simulink model "newQuatLib"  (R2015a)
settings: Solver=ode45  StartTime=0.0  StopTime=10.0  RelTol=1e-3
undefined symbols (not defined in the file): randquatiso
libraries: simulink x1
(part 1 of 2)
settings Model: Creator=lagadec  LastModifiedBy=lagadec
settings DebuggingCC: UnderspecifiedInitializationDetection=Classic  MergeDetectMultiDrivingBlocksExec=none  SolverPrmCheckMsg=warning

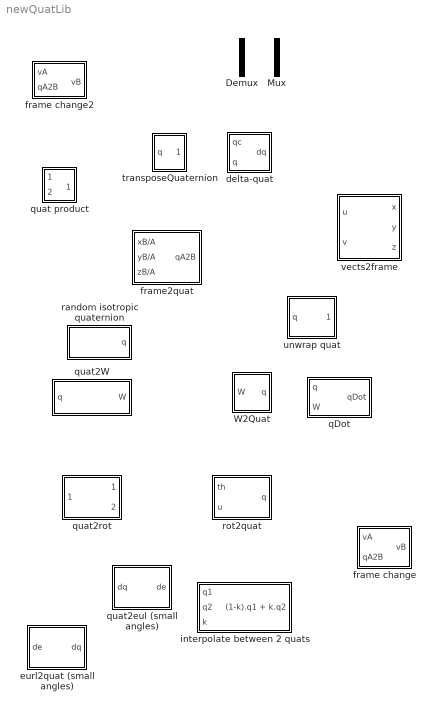
== system newQuatLib ==
  Demux : Demux  Outputs=[1 3]
  Mux : Mux  Inputs=2
  W2Quat : Subsystem  Tag=40  mask(W2Quat){q_init=randquatiso(1)}
      mask prompts: q_init "Initial quaternion"
      mask help:
      | Compute attitude quaternion from instantaneous angular velocity of the rigid body expressed in body frame :
      | w = [p q r]'
      |
      | K. Lagadec 1998
      mask Help: eval('AstrolibHelp');
      mask Display: disp('\Omega=\intq','texmode','on')
  delta-quat : Subsystem  mask(deltaQuaternion){}
      mask help:
      | Computes the 'difference' between 2 attitudes, i.e. the quaternion Dq such that:
      | dq = qc'*q
      | (analogous to dtheta = theta_c - theta for 1-d angles)
  eurl2quat (small angles) : Subsystem  mask(Small euler angles error to small quat){}
      mask help: dq = [1; e(1)/2 ; e(2)/2 ; e(3)/2]
  frame change : Subsystem  mask(Frame change){inLabel=I, outLabel=B}
      mask prompts: inLabel "Label for initial frame"; outLabel "Label for target frame"
      mask help: Express input vector in frame B, using the quaternion describing the rotation from frame A to frame B.
      mask Display:
      | port_label('input',1,['v',inLabel]);
      | port_label('output',1,['v',outLabel]);
      | port_label('input',2,['q',inLabel,'2',outLabel]);
  frame change2 : Subsystem  mask(Frame change){inLabel=I, outLabel=T, flipQuat=off}
      mask prompts: inLabel "Label for initial frame"; outLabel "Label for target frame"; flipQuat "Transpose input quaternion"
      mask help: Express input vector in target frame, using the quaternion describing the rotation from origin frame to target frame.
      mask init:
      | if flipQuat
      |     qLabel = ['q',outLabel,'2',inLabel];
      | else
      |     qLabel = ['q',inLabel,'2',outLabel];
      | end
      mask Display:
      | port_label('input',1,['v',inLabel]);
      | port_label('output',1,['v',outLabel]);
      | port_label('input',2,qLabel);
  frame2quat : Subsystem  mask(Compute quaternion from 3 orthogonal unit vectors){Alabel=I, Blabel=B}
      mask prompts: Alabel "Label for origin frame"; Blabel "Label for target frame"
      mask help: Determines the attitude quaternion representing the rotation which transforms the origin frame into the target frame, from the unit vectors of target frame expressed in origin frame.
      mask Display:
      | port_label('input',1,['x',Blabel,'/',Alabel]);
      | port_label('input',2,['y',Blabel,'/',Alabel]);
      | port_label('input',3,['z',Blabel,'/',Alabel]);
      | port_label('output',1,['q',Alabel,'2',Blabel]);
  interpolate between 2 quats : Subsystem
  qDot : Subsystem  Tag=40  mask(W2dqdt){}
      mask help:
      | Compute quaternion derivative from instantaneous angular velocity of the rigid body expressed in body frame :
      | dq/dt = 0.5*q*W
      | K. Lagadec 1998
  quat product : Subsystem
      mask Display:
      | plot(0.5+cos(linspace(0,2*pi,65))*0.25,0.5+sin(linspace(0,2*pi,65))*0.25);
      | plot([.32 .68],[.32 .68]);
      | plot([.68 .32],[.32 .68]);
  quat2W : Subsystem  mask(Quaternion differentiation){Ts=1}
      mask prompts: Ts "Sample time"
      mask help:
      | Compute angular velocity vector by differentiating the attitude quaternion :
      |
      | W = 2*q'*dq/dt
      mask Display: disp('\Omega~2q''(\deltaq/\deltat)','texmode','on')
  quat2eul (small angles) : Subsystem  mask(Small quat error to small angles error){}
      mask help:
      | [dphi,dtheta,dpsi] = u*dTheta
      | where
      | dq = [cos(dTheta/2); u*sin(dTheta/2)]
  quat2rot : Subsystem  mask(Find axis and angle from quaternion){Alabel=I, Blabel=B}
      mask prompts: Alabel "Label for origin frame"; Blabel "Label for target frame"
      mask help: Extracts the axis (unit vector) and angle (rad) of the rotation from origin frame to target frame, from the quaternion representing that rotation
      mask Display:
      | port_label('input',1,['q',Alabel,'2',Blabel]);
      | port_label('output',1,['th_',Alabel,'2',Blabel]);
      | port_label('output',2,['u_',Alabel]);
  random isotropic quaternion : Subsystem  mask(Random quaternion (isotropic)){Ts=1}
      mask prompts: Ts "Sample time"
      mask help:
      | Simple random isotropic quaternion, made by normalizing a 4-vector with gaussian random components.
      | (because quaternion space is equivalent to the 3-sphere (unit sphere in 4D)).
      |
      | K. Lagadec, 2016
      mask Display: disp('randquat')
  rot2quat : Subsystem  mask(Rotation to quaternion){Alabel=I, Blabel=B}
      mask prompts: Alabel "Label for origin frame"; Blabel "Label for target frame"
      mask help:
      | Computes quaternion from elementary components: rotation axis u and rotation angle theta
      | by convention, norm(u) = 1
      | q(1) = cos(theta/2)
      | q(2) = u(1)*sin(theta/2)
      | q(3) = u(2)*sin(theta/2)
      | q(4) = u(3)*sin(theta/2)
      |
      | K. Lagadec 2000
      mask Display:
      | port_label('output',1,['q',Alabel,'2',Blabel]);
      | port_label('input',1,['th_',Alabel,'2',Blabel]);
      | port_label('input',2,['u_',Alabel]);
  transposeQuaternion : Subsystem  mask(transposeQuaternion){}
      mask help:
      | Compute the transpose (inverse or conjugate) of the input quaternion
      |
      | Inputs:
      |   q     Quaternion
      |
      | Outputs:
      |   qt     Transpose of the input quaternion
      mask Help: eval('starDoc simulink/transposeQuaternion');
      mask Display: disp('q''');
  unwrap quat : Subsystem  mask(Unwrap quaternion){}
      mask help: Avoid sudden jumps q => -q when both quaternions are equivalent. Produces smooth quaternion output unless there are real discontinuities in attitude.
  vects2frame : Subsystem  mask(vects2frame){axisOrder=yx}
      mask prompts: axisOrder "Axes defined by u and v"
      mask help:
      | Construct a right-handed orthogonal frame from 2 directions
      | The first direction defines one of the target axes
      | The second direction defines another axis
      | If the two directions are not perpendicular, the first one has priority.
      | If the two directions are parallel, there will be a div by zero.
      |
      | Input vectors are normalized inside the mask
      mask init:
      | switch axisOrder
      |     case 'xy'
      |         order_i = [1 2 3];
      |         sign_i = [1 1 1];
      |     case 'xz'
      |         order_i = [1 3 2];
      |         sign_i = [1 -1 1];
      |     case 'yx'
      |         order_i = [2 1 3];
      |         sign_i = [1 1 -1];
      |     case 'yz'
      |         order_i = [3 1 2];
      |         sign_i = [1 1 1];
      |     case 'zx'
      |         order_i = [2 3 1];
      |         sign_i = [1 1 1];
      |     case 'zy'
      |         order_i = [3 2 1];
      |         sign_i = [-1 1 1];
      | end
      mask TypeOptions axisOrder: xy | xz | yx | yz | zx | zy
      mask Display:
      | port_label('input',1,axisOrder(1));
      | port_label('input',2,axisOrder(2));
      | 
      | port_label('output',1,'x');
      | port_label('output',2,'y');
      | port_label('output',3,'z');

== system newQuatLib/W2Quat ==
  note: q_dot = 1/2 q.W
  W : Inport  PortDimensions=3
  Constant : Constant  Value=0
  Gain : Gain  Gain=1/2  SaturateOnIntegerOverflow=on  OutDataTypeStr=Inherit: Same as input  ParamDataTypeStr=Inherit: Same as input
  Integrator : Integrator  InitialCondition=q_init
  Normalization : Subsystem  Tag=74
      mask help:
      | normalizes a vector, so that the output is a unit vector.
      | y = u/||u||
      mask Help: eval('AstrolibHelp');
      mask Display: disp('X/||X||');
  Transform into quaternion : Mux  Inputs=2
  quat product : Subsystem
      mask Display:
      | plot(0.5+cos(linspace(0,2*pi,65))*0.3,0.5+sin(linspace(0,2*pi,65))*0.3);
      | plot([.29 .71],[.29 .71]);
      | plot([.71 .29],[.29 .71]);
  q : Outport  PortDimensions=4  InitialOutput=0
  wires:
  quat product/1(q1*q2) -> Gain/1
  Gain/1 -> Integrator/1  "q_dot"
  Integrator/1 -> Normalization/1(X)
  Normalization/1(X/||X||) -> quat product/1(q1), q/1
  Transform into quaternion/1 -> quat product/2(q2)
  W/1 -> Transform into quaternion/2
  Constant/1 -> Transform into quaternion/1

== system newQuatLib/delta-quat ==
  qc : Inport  PortDimensions=4
  q : Inport  Port=2  PortDimensions=4
  quat product : Subsystem
      mask Display:
      | plot(0.5+cos(linspace(0,2*pi,65))*0.3,0.5+sin(linspace(0,2*pi,65))*0.3);
      | plot([.29 .71],[.29 .71]);
      | plot([.71 .29],[.29 .71]);
  transposeQuaternion : Subsystem  mask(transposeQuaternion){}
      mask help:
      | Compute the transpose (inverse or conjugate) of the input quaternion
      |
      | Inputs:
      |   q     Quaternion
      |
      | Outputs:
      |   qt     Transpose of the input quaternion
      mask Help: eval('starDoc simulink/transposeQuaternion');
      mask Display: disp('q''');
  dq : Outport  PortDimensions=4
  wires:
  q/1 -> quat product/2(q2)
  quat product/1(q1*q2) -> dq/1
  qc/1 -> transposeQuaternion/1(q)
  transposeQuaternion/1(q') -> quat product/1(q1)  "qA2B"

== system newQuatLib/eurl2quat (small angles) ==
  de : Inport  PortDimensions=3
  Mux : Mux  Inputs=2
  Normalization : Subsystem  Tag=74
      mask help:
      | normalizes a vector, so that the output is a unit vector.
      | y = u/||u||
      mask Help: eval('AstrolibHelp');
      mask Display: disp('X/||X||');
  half : Gain  Gain=0.5
  scalar : Constant
  dq : Outport  PortDimensions=4
  wires:
  de/1 -> half/1
  half/1 -> Mux/2
  scalar/1 -> Mux/1
  Mux/1 -> Normalization/1(X)
  Normalization/1(X/||X||) -> dq/1

== system newQuatLib/frame change ==
  vA : Inport
  qA2B : Inport  Port=2
  Constant : Constant
  Demux : Demux  Outputs=[1 3]
  Mux : Mux  Inputs=2
  Product : Product  Inputs=/*  SaturateOnIntegerOverflow=on  OutDataTypeStr=Inherit: Same as first input
  quat product : Subsystem
      mask Display:
      | plot(0.5+cos(linspace(0,2*pi,65))*0.3,0.5+sin(linspace(0,2*pi,65))*0.3);
      | plot([.29 .71],[.29 .71]);
      | plot([.71 .29],[.29 .71]);
  quat product1 : Subsystem
      mask Display:
      | plot(0.5+cos(linspace(0,2*pi,65))*0.3,0.5+sin(linspace(0,2*pi,65))*0.3);
      | plot([.29 .71],[.29 .71]);
      | plot([.71 .29],[.29 .71]);
  transposeQuaternion : Subsystem  mask(transposeQuaternion){}
      mask help:
      | Compute the transpose (inverse or conjugate) of the input quaternion
      |
      | Inputs:
      |   q     Quaternion
      |
      | Outputs:
      |   qt     Transpose of the input quaternion
      mask Help: eval('starDoc simulink/transposeQuaternion');
      mask Display: disp('q''');
  vB : Outport
  wires:
  Product/1 -> vB/1
  quat product1/1(q1*q2) -> Demux/1
  quat product/1(q1*q2) -> quat product1/1(q1)
  Mux/1 -> quat product/2(q2)
  transposeQuaternion/1(q') -> quat product/1(q1)
  qA2B/1 -> quat product1/2(q2), transposeQuaternion/1(q)
  vA/1 -> Mux/2
  Constant/1 -> Mux/1
  Demux/1 -> Product/1
  Demux/2 -> Product/2

== system newQuatLib/frame change2 ==
  vA : Inport  PortDimensions=3
  qA2B : Inport  Port=2  PortDimensions=4
  Constant : Constant
  Constant1 : Constant  Value=not(flipQuat)
  Constant2 : Constant  Value=flipQuat
  Demux : Demux  Outputs=[1 3]
  Mux : Mux  Inputs=2
  Product : Product  Inputs=/*  SaturateOnIntegerOverflow=on  OutDataTypeStr=Inherit: Same as first input
  Switch : Switch  Criteria=u2 ~= 0
  Switch1 : Switch  Criteria=u2 ~= 0
  quat product : Subsystem
      mask Display:
      | plot(0.5+cos(linspace(0,2*pi,65))*0.3,0.5+sin(linspace(0,2*pi,65))*0.3);
      | plot([.29 .71],[.29 .71]);
      | plot([.71 .29],[.29 .71]);
  quat product1 : Subsystem
      mask Display:
      | plot(0.5+cos(linspace(0,2*pi,65))*0.3,0.5+sin(linspace(0,2*pi,65))*0.3);
      | plot([.29 .71],[.29 .71]);
      | plot([.71 .29],[.29 .71]);
  transposeQuaternion : Subsystem  mask(transposeQuaternion){}
      mask help:
      | Compute the transpose (inverse or conjugate) of the input quaternion
      |
      | Inputs:
      |   q     Quaternion
      |
      | Outputs:
      |   qt     Transpose of the input quaternion
      mask Help: eval('starDoc simulink/transposeQuaternion');
      mask Display: disp('q''');
  vB : Outport  PortDimensions=3
  wires:
  Demux/2 -> Product/2
  Demux/1 -> Product/1
  Constant/1 -> Mux/1
  vA/1 -> Mux/2
  qA2B/1 -> transposeQuaternion/1(q), Switch/3, Switch1/3
  transposeQuaternion/1(q') -> Switch1/1, Switch/1
  Mux/1 -> quat product/2(q2)
  quat product/1(q1*q2) -> quat product1/1(q1)
  quat product1/1(q1*q2) -> Demux/1
  Product/1 -> vB/1
  Constant1/1 -> Switch/2
  Switch/1 -> quat product/1(q1)
  Constant2/1 -> Switch1/2
  Switch1/1 -> quat product1/2(q2)

== system newQuatLib/frame2quat ==
  xB/A : Inport  PortDimensions=3
  yB/A : Inport  Port=2  PortDimensions=3
  zB/A : Inport  Port=3  PortDimensions=3
  MATLAB Function : MATLAB Function  TreatAsAtomicUnit=on
  qA2B : Outport  PortDimensions=4
  wires:
  xB/A/1 -> MATLAB Function/1(xB)
  yB/A/1 -> MATLAB Function/2(yB)
  zB/A/1 -> MATLAB Function/3(zB)
  MATLAB Function/1(qA2B) -> qA2B/1

== system newQuatLib/interpolate between 2 quats ==
  q1 : Inport
  q2 : Inport  Port=2
  k : Inport  Port=3
  MATLAB Function : MATLAB Function  TreatAsAtomicUnit=on
  (1-k).q1 + k.q2 : Outport
  wires:
  MATLAB Function/1(qi) -> (1-k).q1 + k.q2/1
  q2/1 -> MATLAB Function/2(q2)
  q1/1 -> MATLAB Function/1(q1)
  k/1 -> MATLAB Function/3(k)

== system newQuatLib/qDot ==
  note: q_dot = 1/2 q.W
  q : Inport  PortDimensions=4
  W : Inport  Port=2  PortDimensions=3
  Constant : Constant  Value=0
  Gain : Gain  Gain=1/2  SaturateOnIntegerOverflow=on  OutDataTypeStr=Inherit: Same as input  ParamDataTypeStr=Inherit: Same as input
  Transform into quaternion : Mux  Inputs=2
  quat product : Subsystem
      mask Display:
      | plot(0.5+cos(linspace(0,2*pi,65))*0.3,0.5+sin(linspace(0,2*pi,65))*0.3);
      | plot([.29 .71],[.29 .71]);
      | plot([.71 .29],[.29 .71]);
  qDot : Outport  PortDimensions=4  InitialOutput=0
  wires:
  Constant/1 -> Transform into quaternion/1
  W/1 -> Transform into quaternion/2
  Transform into quaternion/1 -> quat product/2(q2)
  quat product/1(q1*q2) -> Gain/1
  Gain/1 -> qDot/1  "q_dot"
  q/1 -> quat product/1(q1)

== system newQuatLib/quat product ==
  q1 : Inport  PortDimensions=4
  q2 : Inport  Port=2  PortDimensions=4
  Cross Product : Subsystem  Tag=68  mask(CrossProduct){}
      mask help: Compute the cross product of two 3-vectors : y = u1 x u2
      mask Display:
      | plot([.4 .6],[.4 .6]);
      | plot([.6 .4],[.4 .6]);
  Demux : Demux  Outputs=[1 3]
  Demux1 : Demux  Outputs=[1 3]
  Dot Product : DotProduct  InputSameDT=on  OutDataTypeStr=Inherit: Inherit via internal rule
  Mux : Mux  Inputs=2
  Product : Product  SaturateOnIntegerOverflow=on  OutDataTypeStr=Inherit: Same as first input
  Product1 : Product  SaturateOnIntegerOverflow=on  OutDataTypeStr=Inherit: Same as first input
  Product2 : Product  SaturateOnIntegerOverflow=on  OutDataTypeStr=Inherit: Same as first input
  Sum : Sum  Inputs=+++  SaturateOnIntegerOverflow=on
  Sum1 : Sum  Inputs=|+-  SaturateOnIntegerOverflow=on
  q1*q2 : Outport  PortDimensions=4
  wires:
  Demux/2 -> Product1/2, Cross Product/1(u1), Dot Product/2
  Demux/1 -> Product/1, Product2/1
  Demux1/1 -> Product1/1, Product2/2
  Demux1/2 -> Cross Product/2(u2), Product/2, Dot Product/1
  Cross Product/1(u1xu2) -> Sum/2
  Product/1 -> Sum/1
  Product1/1 -> Sum/3
  Sum/1 -> Mux/2  "vector"
  Product2/1 -> Sum1/1
  Dot Product/1 -> Sum1/2
  Sum1/1 -> Mux/1  "scalar"
  q1/1 -> Demux/1
  Mux/1 -> q1*q2/1
  q2/1 -> Demux1/1

== system newQuatLib/quat2W ==
  note: W = 2*q'*dq/dt
  q : Inport  PortDimensions=4  SampleTime=Ts
  Discrete Derivative : simulink/Discrete/Discrete Derivative  gainval=1.0  ICPrevScaledInput=0.0  InputProcessing=Inherited  OutMin=[]  OutMax=[]  OutDataType=fixdt(1, 16)  OutScaling=2^-10  DoSatur=off
  Selector : Selector  InputPortWidth=4  Indices=[2:4]
  quat product : Subsystem
      mask Display:
      | plot(0.5+cos(linspace(0,2*pi,65))*0.25,0.5+sin(linspace(0,2*pi,65))*0.25);
      | plot([.32 .68],[.32 .68]);
      | plot([.68 .32],[.32 .68]);
  times two : Gain  Gain=2
  transposeQuaternion : Subsystem  mask(transposeQuaternion){}
      mask help:
      | Compute the transpose (inverse or conjugate) of the input quaternion
      |
      | Inputs:
      |   q     Quaternion
      |
      | Outputs:
      |   qt     Transpose of the input quaternion
      mask Help: eval('starDoc simulink/transposeQuaternion');
      mask Display: disp('q''');
  unwrap quat : Subsystem  mask(Unwrap quaternion){}
      mask help: Avoid sudden jumps q => -q when both quaternions are equivalent. Produces smooth quaternion output unless there are real discontinuities in attitude.
  W : Outport  PortDimensions=3
  wires:
  q/1 -> unwrap quat/1(q)
  times two/1 -> W/1
  Selector/1 -> times two/1
  quat product/1(q1*q2) -> Selector/1
  Discrete Derivative/1 -> quat product/2(q2)  "scalar"
  unwrap quat/1(q_unw) -> Discrete Derivative/1, transposeQuaternion/1(q)
  transposeQuaternion/1(q') -> quat product/1(q1)

== system newQuatLib/quat2eul (small angles) ==
  dq : Inport  PortDimensions=4
  Demux : Demux  Outputs=[1 3]
  Gain : Gain  Gain=2
  manage quat sign : Switch  Criteria=u2 > Threshold
  take opposite : Gain  Gain=-1
  de : Outport  PortDimensions=3
  wires:
  Gain/1 -> de/1
  dq/1 -> Demux/1
  Demux/1 -> manage quat sign/2  "scalar"
  Demux/2 -> manage quat sign/1, take opposite/1
  take opposite/1 -> manage quat sign/3
  manage quat sign/1 -> Gain/1

== system newQuatLib/quat2rot ==
  q_AB : Inport  PortDimensions=4
  Constant : Constant
  Demux : Demux  Outputs=[1 3]
  Divide : Product  Inputs=***
  Divide1 : Product  Inputs=/
  Divide2 : Product  Inputs=**
  Gain : Gain  Gain=2
  Norm : Subsystem  mask(Norm){}
      mask help: Computes the norm of a vector : y = ||u||.
      mask Help: eval('AstrolibHelp');
      mask Display: disp('||X||');
  Sign : Signum  ZeroCross=off
  Switch : Switch  Criteria=u2 ~= 0  ZeroCross=off
  Trigonometric Function : Trigonometry  Operator=atan2
  angleB2A : Outport  PortDimensions=1
  vector_A : Outport  Port=2  PortDimensions=3
  wires:
  Sign/1 -> Divide2/2, Divide/1
  Divide2/1 -> Trigonometric Function/2
  Divide1/1 -> Divide/3
  q_AB/1 -> Demux/1
  Demux/1 -> Divide2/1, Sign/1
  Demux/2 -> Norm/1(X), Divide/2
  Trigonometric Function/1 -> Gain/1
  Gain/1 -> angleB2A/1
  Divide/1 -> vector_A/1
  Norm/1(||X||) -> Trigonometric Function/1, Switch/1, Switch/2
  Switch/1 -> Divide1/1
  Constant/1 -> Switch/3

== system newQuatLib/random isotropic quaternion ==
  Normalization : Subsystem  Tag=74
      mask help:
      | normalizes a vector, so that the output is a unit vector.
      | y = u/||u||
      mask Help: eval('AstrolibHelp');
      mask Display: disp('X/||X||');
  Random Number : RandomNumber  Seed=ceil(rand(4,1)*10000)  SampleTime=Ts
  q : Outport
  wires:
  Normalization/1(X/||X||) -> q/1  "q"
  Random Number/1 -> Normalization/1(X)

== system newQuatLib/rot2quat ==
  note: q(1) = cos(theta/2)
      | q(2) = u(1)*sin(theta/2)
      | q(3) = u(2)*sin(theta/2)
      | q(4) = u(3)*sin(theta/2)
  th : Inport  PortDimensions=1
  u : Inport  Port=2  PortDimensions=3
  Gain1 : Gain  Gain=1/2  SaturateOnIntegerOverflow=on  OutDataTypeStr=Inherit: Same as input  ParamDataTypeStr=Inherit: Same as input
  Mux : Mux  Inputs=2
  Product : Product  SaturateOnIntegerOverflow=on  RndMeth=Zero  InputSameDT=on  OutDataTypeStr=Inherit: Same as first input
  Trigonometric Function1 : Trigonometry
  Trigonometric Function2 : Trigonometry  Operator=cos
  q : Outport  PortDimensions=4
  wires:
  u/1 -> Product/2
  Trigonometric Function1/1 -> Product/1
  Mux/1 -> q/1
  Gain1/1 -> Trigonometric Function2/1, Trigonometric Function1/1
  th/1 -> Gain1/1
  Product/1 -> Mux/2
  Trigonometric Function2/1 -> Mux/1

== system newQuatLib/transposeQuaternion ==
  q : Inport  PortDimensions=4
  Gain1 : Gain  Gain=[1 -1 -1 -1]  SaturateOnIntegerOverflow=on  OutDataTypeStr=Inherit: Same as input  ParamDataTypeStr=Inherit: Same as input
  q' : Outport  PortDimensions=4
  wires:
  q/1 -> Gain1/1
  Gain1/1 -> q'/1

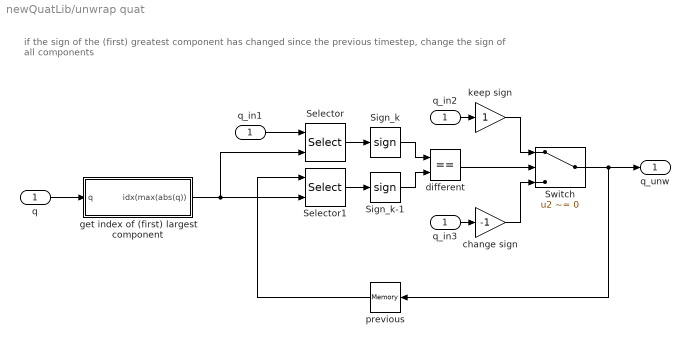
== system newQuatLib/unwrap quat ==
  note: if the sign of the (first) greatest component has changed since the previous timestep, change the sign of all components
  q : Inport
  Selector : Selector  InputPortWidth=4  IndexOptions=Index vector (port)  Indices=[1 3]
  Selector1 : Selector  InputPortWidth=4  IndexOptions=Index vector (port)  Indices=[1 3]
  Sign_k : Signum
  Sign_k-1 : Signum
  Switch : Switch  Criteria=u2 ~= 0
  change sign : Gain  Gain=-1
  different : RelationalOperator  Operator===  OutDataTypeStr=boolean
  get index of (first) largest component : Subsystem
  keep sign : Gain
  previous : Memory  X0=[1 1 1 1]  InheritSampleTime=on
  q_in1 : InportShadow
  q_in2 : InportShadow
  q_in3 : InportShadow
  q_unw : Outport
  wires:
  q_in3/1 -> change sign/1
  change sign/1 -> Switch/3
  keep sign/1 -> Switch/1
  q_in2/1 -> keep sign/1
  different/1 -> Switch/2
  Sign_k/1 -> different/1
  Sign_k-1/1 -> different/2
  Selector/1 -> Sign_k/1
  q_in1/1 -> Selector/1
  Switch/1 -> q_unw/1, previous/1
  previous/1 -> Selector1/1
  Selector1/1 -> Sign_k-1/1
  get index of (first) largest component/1(idx(max(abs(q))) -> Selector/2, Selector1/2
  q/1 -> get index of (first) largest component/1(q)

== system newQuatLib/vects2frame ==
  u : Inport  PortDimensions=3
  v : Inport  Port=2  PortDimensions=3
  Normalization : Subsystem  Tag=74
      mask help:
      | normalizes a vector, so that the output is a unit vector.
      | y = u/||u||
      mask Help: eval('AstrolibHelp');
      mask Display: disp('X/||X||');
  Normalization1 : Subsystem  Tag=74
      mask help:
      | normalizes a vector, so that the output is a unit vector.
      | y = u/||u||
      mask Help: eval('AstrolibHelp');
      mask Display: disp('X/||X||');
  cross product : Subsystem  Tag=68  mask(CrossProduct){}
      mask help: Compute the cross product of two 3-vectors : y = u1 x u2
      mask Display:
      | plot([.4 .6],[.4 .6]);
      | plot([.6 .4],[.4 .6]);
  cross product1 : Subsystem  Tag=68  mask(CrossProduct){}
      mask help: Compute the cross product of two 3-vectors : y = u1 x u2
      mask Display:
      | plot([.4 .6],[.4 .6]);
      | plot([.6 .4],[.4 .6]);
  reorder : Subsystem
  x : Outport
  y : Outport  Port=2
  z : Outport  Port=3
  wires:
  reorder/3(z) -> z/1
  reorder/2(y) -> y/1
  reorder/1(x) -> x/1
  cross product1/1(u1xu2) -> reorder/2((uxv)xu)
  Normalization1/1(X/||X||) -> cross product1/1(u1), reorder/3(uxv)
  cross product/1(u1xu2) -> Normalization1/1(X)
  v/1 -> cross product/2(u2)
  Normalization/1(X/||X||) -> cross product1/2(u2), reorder/1(u)
  u/1 -> Normalization/1(X), cross product/1(u1)

== system newQuatLib/W2Quat/Normalization ==
  X : Inport
      settings: AttributesFormatString=(#%<Tag>)
      mask Help: eval('AstrolibHelp');
  Constant : Constant
  Norm : Subsystem  mask(Norm){}
      mask help: Computes the norm of a vector : y = ||u||.
      settings: AttributesFormatString=(#%<Tag>)
      mask Help: eval('AstrolibHelp');
      mask Display: disp('||X||');
  Product : Product  Inputs=*/  RndMeth=Zero
  avoid div by zero : Switch  Criteria=u2 ~= 0
  x(1) = 1 : Assignment  DiagnosticForDimensions=Warning
  X/||X|| : Outport  InitialOutput=0
      settings: AttributesFormatString=(#%<Tag>)
      mask Help: eval('AstrolibHelp');
  wires:
  Norm/1(||X||) -> Product/2, avoid div by zero/2
  X/1 -> Product/1, x(1) = 1/1, Norm/1(X)
  Product/1 -> avoid div by zero/1
  avoid div by zero/1 -> X/||X||/1
  x(1) = 1/1 -> avoid div by zero/3
  Constant/1 -> x(1) = 1/2

== system newQuatLib/W2Quat/quat product ==
  q1 : Inport
  q2 : Inport  Port=2
  Cross Product : Subsystem  Tag=68  mask(CrossProduct){}
      mask help: Compute the cross product of two 3-vectors : y = u1 x u2
      mask Display:
      | plot([.4 .6],[.4 .6]);
      | plot([.6 .4],[.4 .6]);
  Demux : Demux  Outputs=[1 3]
  Demux1 : Demux  Outputs=[1 3]
  Dot Product : DotProduct  InputSameDT=on  OutDataTypeStr=Inherit: Inherit via internal rule
  Mux : Mux  Inputs=2
  Product : Product  SaturateOnIntegerOverflow=on  OutDataTypeStr=Inherit: Same as first input
  Product1 : Product  SaturateOnIntegerOverflow=on  OutDataTypeStr=Inherit: Same as first input
  Product2 : Product  SaturateOnIntegerOverflow=on  OutDataTypeStr=Inherit: Same as first input
  Sum : Sum  Inputs=+++  SaturateOnIntegerOverflow=on
  Sum1 : Sum  Inputs=|+-  SaturateOnIntegerOverflow=on
  q1*q2 : Outport
  wires:
  Demux/2 -> Product1/2, Cross Product/1(u1), Dot Product/2
  Demux/1 -> Product/1, Product2/1
  Demux1/1 -> Product1/1, Product2/2
  Demux1/2 -> Cross Product/2(u2), Product/2, Dot Product/1
  Cross Product/1(u1xu2) -> Sum/2
  Product/1 -> Sum/1
  Product1/1 -> Sum/3
  Sum/1 -> Mux/2  "vector"
  Product2/1 -> Sum1/1
  Dot Product/1 -> Sum1/2
  Sum1/1 -> Mux/1  "scalar"
  q1/1 -> Demux/1
  Mux/1 -> q1*q2/1
  q2/1 -> Demux1/1

== system newQuatLib/delta-quat/quat product ==
  q1 : Inport
  q2 : Inport  Port=2
  Cross Product : Subsystem  Tag=68  mask(CrossProduct){}
      mask help: Compute the cross product of two 3-vectors : y = u1 x u2
      mask Display:
      | plot([.4 .6],[.4 .6]);
      | plot([.6 .4],[.4 .6]);
  Demux : Demux  Outputs=[1 3]
  Demux1 : Demux  Outputs=[1 3]
  Dot Product : DotProduct  InputSameDT=on  OutDataTypeStr=Inherit: Inherit via internal rule
  Mux : Mux  Inputs=2
  Product : Product  SaturateOnIntegerOverflow=on  OutDataTypeStr=Inherit: Same as first input
  Product1 : Product  SaturateOnIntegerOverflow=on  OutDataTypeStr=Inherit: Same as first input
  Product2 : Product  SaturateOnIntegerOverflow=on  OutDataTypeStr=Inherit: Same as first input
  Sum : Sum  Inputs=+++  SaturateOnIntegerOverflow=on
  Sum1 : Sum  Inputs=|+-  SaturateOnIntegerOverflow=on
  q1*q2 : Outport
  wires:
  Demux/2 -> Product1/2, Cross Product/1(u1), Dot Product/2
  Demux/1 -> Product/1, Product2/1
  Demux1/1 -> Product1/1, Product2/2
  Demux1/2 -> Cross Product/2(u2), Product/2, Dot Product/1
  Cross Product/1(u1xu2) -> Sum/2
  Product/1 -> Sum/1
  Product1/1 -> Sum/3
  Sum/1 -> Mux/2  "vector"
  Product2/1 -> Sum1/1
  Dot Product/1 -> Sum1/2
  Sum1/1 -> Mux/1  "scalar"
  q1/1 -> Demux/1
  Mux/1 -> q1*q2/1
  q2/1 -> Demux1/1

== system newQuatLib/delta-quat/transposeQuaternion ==
  q : Inport
  Gain1 : Gain  Gain=[1 -1 -1 -1]  SaturateOnIntegerOverflow=on  OutDataTypeStr=Inherit: Same as input  ParamDataTypeStr=Inherit: Same as input
  q' : Outport
  wires:
  q/1 -> Gain1/1
  Gain1/1 -> q'/1

== system newQuatLib/eurl2quat (small angles)/Normalization ==
  X : Inport
      settings: AttributesFormatString=(#%<Tag>)
      mask Help: eval('AstrolibHelp');
  Constant : Constant
  Norm : Subsystem  mask(Norm){}
      mask help: Computes the norm of a vector : y = ||u||.
      settings: AttributesFormatString=(#%<Tag>)
      mask Help: eval('AstrolibHelp');
      mask Display: disp('||X||');
  Product : Product  Inputs=*/  RndMeth=Zero
  avoid div by zero : Switch  Criteria=u2 ~= 0
  x(1) = 1 : Assignment  DiagnosticForDimensions=Warning
  X/||X|| : Outport  InitialOutput=0
      settings: AttributesFormatString=(#%<Tag>)
      mask Help: eval('AstrolibHelp');
  wires:
  Norm/1(||X||) -> Product/2, avoid div by zero/2
  X/1 -> Product/1, x(1) = 1/1, Norm/1(X)
  Product/1 -> avoid div by zero/1
  avoid div by zero/1 -> X/||X||/1
  x(1) = 1/1 -> avoid div by zero/3
  Constant/1 -> x(1) = 1/2

== system newQuatLib/frame change/quat product ==
  q1 : Inport
  q2 : Inport  Port=2
  Cross Product : Subsystem  Tag=68  mask(CrossProduct){}
      mask help: Compute the cross product of two 3-vectors : y = u1 x u2
      mask Display:
      | plot([.4 .6],[.4 .6]);
      | plot([.6 .4],[.4 .6]);
  Demux : Demux  Outputs=[1 3]
  Demux1 : Demux  Outputs=[1 3]
  Dot Product : DotProduct  InputSameDT=on  OutDataTypeStr=Inherit: Inherit via internal rule
  Mux : Mux  Inputs=2
  Product : Product  SaturateOnIntegerOverflow=on  OutDataTypeStr=Inherit: Same as first input
  Product1 : Product  SaturateOnIntegerOverflow=on  OutDataTypeStr=Inherit: Same as first input
  Product2 : Product  SaturateOnIntegerOverflow=on  OutDataTypeStr=Inherit: Same as first input
  Sum : Sum  Inputs=+++  SaturateOnIntegerOverflow=on
  Sum1 : Sum  Inputs=|+-  SaturateOnIntegerOverflow=on
  q1*q2 : Outport
  wires:
  Demux/2 -> Product1/2, Cross Product/1(u1), Dot Product/2
  Demux/1 -> Product/1, Product2/1
  Demux1/1 -> Product1/1, Product2/2
  Demux1/2 -> Cross Product/2(u2), Product/2, Dot Product/1
  Cross Product/1(u1xu2) -> Sum/2
  Product/1 -> Sum/1
  Product1/1 -> Sum/3
  Sum/1 -> Mux/2  "vector"
  Product2/1 -> Sum1/1
  Dot Product/1 -> Sum1/2
  Sum1/1 -> Mux/1  "scalar"
  q1/1 -> Demux/1
  Mux/1 -> q1*q2/1
  q2/1 -> Demux1/1

== system newQuatLib/frame change/quat product1 ==
  q1 : Inport
  q2 : Inport  Port=2
  Cross Product : Subsystem  Tag=68  mask(CrossProduct){}
      mask help: Compute the cross product of two 3-vectors : y = u1 x u2
      mask Display:
      | plot([.4 .6],[.4 .6]);
      | plot([.6 .4],[.4 .6]);
  Demux : Demux  Outputs=[1 3]
  Demux1 : Demux  Outputs=[1 3]
  Dot Product : DotProduct  InputSameDT=on  OutDataTypeStr=Inherit: Inherit via internal rule
  Mux : Mux  Inputs=2
  Product : Product  SaturateOnIntegerOverflow=on  OutDataTypeStr=Inherit: Same as first input
  Product1 : Product  SaturateOnIntegerOverflow=on  OutDataTypeStr=Inherit: Same as first input
  Product2 : Product  SaturateOnIntegerOverflow=on  OutDataTypeStr=Inherit: Same as first input
  Sum : Sum  Inputs=+++  SaturateOnIntegerOverflow=on
  Sum1 : Sum  Inputs=|+-  SaturateOnIntegerOverflow=on
  q1*q2 : Outport
  wires:
  q2/1 -> Demux1/1
  Mux/1 -> q1*q2/1
  q1/1 -> Demux/1
  Sum1/1 -> Mux/1  "scalar"
  Dot Product/1 -> Sum1/2
  Product2/1 -> Sum1/1
  Sum/1 -> Mux/2  "vector"
  Product1/1 -> Sum/3
  Product/1 -> Sum/1
  Cross Product/1(u1xu2) -> Sum/2
  Demux1/2 -> Dot Product/1, Product/2, Cross Product/2(u2)
  Demux1/1 -> Product2/2, Product1/1
  Demux/1 -> Product2/1, Product/1
  Demux/2 -> Dot Product/2, Cross Product/1(u1), Product1/2

== system newQuatLib/frame change/transposeQuaternion ==
  q : Inport
  Gain1 : Gain  Gain=[1 -1 -1 -1]  SaturateOnIntegerOverflow=on  OutDataTypeStr=Inherit: Same as input  ParamDataTypeStr=Inherit: Same as input
  q' : Outport
  wires:
  q/1 -> Gain1/1
  Gain1/1 -> q'/1

== system newQuatLib/frame change2/quat product ==
  q1 : Inport
  q2 : Inport  Port=2
  Cross Product : Subsystem  Tag=68  mask(CrossProduct){}
      mask help: Compute the cross product of two 3-vectors : y = u1 x u2
      mask Display:
      | plot([.4 .6],[.4 .6]);
      | plot([.6 .4],[.4 .6]);
  Demux : Demux  Outputs=[1 3]
  Demux1 : Demux  Outputs=[1 3]
  Dot Product : DotProduct  InputSameDT=on  OutDataTypeStr=Inherit: Inherit via internal rule
  Mux : Mux  Inputs=2
  Product : Product  SaturateOnIntegerOverflow=on  OutDataTypeStr=Inherit: Same as first input
  Product1 : Product  SaturateOnIntegerOverflow=on  OutDataTypeStr=Inherit: Same as first input
  Product2 : Product  SaturateOnIntegerOverflow=on  OutDataTypeStr=Inherit: Same as first input
  Sum : Sum  Inputs=+++  SaturateOnIntegerOverflow=on
  Sum1 : Sum  Inputs=|+-  SaturateOnIntegerOverflow=on
  q1*q2 : Outport
  wires:
  q2/1 -> Demux1/1
  Mux/1 -> q1*q2/1
  q1/1 -> Demux/1
  Sum1/1 -> Mux/1  "scalar"
  Dot Product/1 -> Sum1/2
  Product2/1 -> Sum1/1
  Sum/1 -> Mux/2  "vector"
  Product1/1 -> Sum/3
  Product/1 -> Sum/1
  Cross Product/1(u1xu2) -> Sum/2
  Demux1/2 -> Dot Product/1, Product/2, Cross Product/2(u2)
  Demux1/1 -> Product2/2, Product1/1
  Demux/1 -> Product2/1, Product/1
  Demux/2 -> Dot Product/2, Cross Product/1(u1), Product1/2

== system newQuatLib/frame change2/quat product1 ==
  q1 : Inport
  q2 : Inport  Port=2
  Cross Product : Subsystem  Tag=68  mask(CrossProduct){}
      mask help: Compute the cross product of two 3-vectors : y = u1 x u2
      mask Display:
      | plot([.4 .6],[.4 .6]);
      | plot([.6 .4],[.4 .6]);
  Demux : Demux  Outputs=[1 3]
  Demux1 : Demux  Outputs=[1 3]
  Dot Product : DotProduct  InputSameDT=on  OutDataTypeStr=Inherit: Inherit via internal rule
  Mux : Mux  Inputs=2
  Product : Product  SaturateOnIntegerOverflow=on  OutDataTypeStr=Inherit: Same as first input
  Product1 : Product  SaturateOnIntegerOverflow=on  OutDataTypeStr=Inherit: Same as first input
  Product2 : Product  SaturateOnIntegerOverflow=on  OutDataTypeStr=Inherit: Same as first input
  Sum : Sum  Inputs=+++  SaturateOnIntegerOverflow=on
  Sum1 : Sum  Inputs=|+-  SaturateOnIntegerOverflow=on
  q1*q2 : Outport
  wires:
  Demux/2 -> Product1/2, Cross Product/1(u1), Dot Product/2
  Demux/1 -> Product/1, Product2/1
  Demux1/1 -> Product1/1, Product2/2
  Demux1/2 -> Cross Product/2(u2), Product/2, Dot Product/1
  Cross Product/1(u1xu2) -> Sum/2
  Product/1 -> Sum/1
  Product1/1 -> Sum/3
  Sum/1 -> Mux/2  "vector"
  Product2/1 -> Sum1/1
  Dot Product/1 -> Sum1/2
  Sum1/1 -> Mux/1  "scalar"
  q1/1 -> Demux/1
  Mux/1 -> q1*q2/1
  q2/1 -> Demux1/1

== system newQuatLib/frame change2/transposeQuaternion ==
  q : Inport
  Gain1 : Gain  Gain=[1 -1 -1 -1]  SaturateOnIntegerOverflow=on  OutDataTypeStr=Inherit: Same as input  ParamDataTypeStr=Inherit: Same as input
  q' : Outport
  wires:
  Gain1/1 -> q'/1
  q/1 -> Gain1/1

== system newQuatLib/qDot/quat product ==
  q1 : Inport
  q2 : Inport  Port=2
  Cross Product : Subsystem  Tag=68  mask(CrossProduct){}
      mask help: Compute the cross product of two 3-vectors : y = u1 x u2
      mask Display:
      | plot([.4 .6],[.4 .6]);
      | plot([.6 .4],[.4 .6]);
  Demux : Demux  Outputs=[1 3]
  Demux1 : Demux  Outputs=[1 3]
  Dot Product : DotProduct  InputSameDT=on  OutDataTypeStr=Inherit: Inherit via internal rule
  Mux : Mux  Inputs=2
  Product : Product  SaturateOnIntegerOverflow=on  OutDataTypeStr=Inherit: Same as first input
  Product1 : Product  SaturateOnIntegerOverflow=on  OutDataTypeStr=Inherit: Same as first input
  Product2 : Product  SaturateOnIntegerOverflow=on  OutDataTypeStr=Inherit: Same as first input
  Sum : Sum  Inputs=+++  SaturateOnIntegerOverflow=on
  Sum1 : Sum  Inputs=|+-  SaturateOnIntegerOverflow=on
  q1*q2 : Outport
  wires:
  q2/1 -> Demux1/1
  Mux/1 -> q1*q2/1
  q1/1 -> Demux/1
  Sum1/1 -> Mux/1  "scalar"
  Dot Product/1 -> Sum1/2
  Product2/1 -> Sum1/1
  Sum/1 -> Mux/2  "vector"
  Product1/1 -> Sum/3
  Product/1 -> Sum/1
  Cross Product/1(u1xu2) -> Sum/2
  Demux1/2 -> Dot Product/1, Product/2, Cross Product/2(u2)
  Demux1/1 -> Product2/2, Product1/1
  Demux/1 -> Product2/1, Product/1
  Demux/2 -> Dot Product/2, Cross Product/1(u1), Product1/2

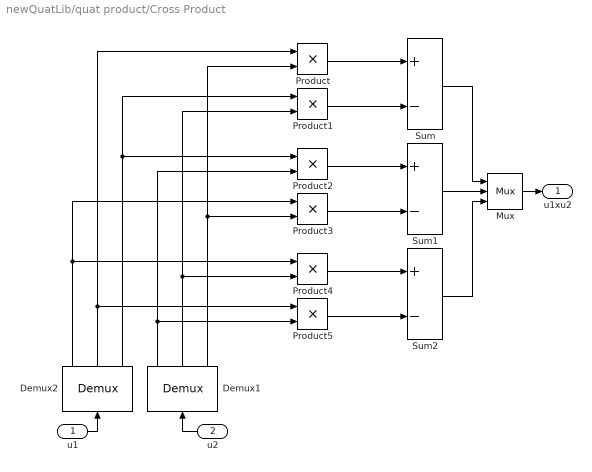
== system newQuatLib/quat product/Cross Product ==
  u1 : Inport
  u2 : Inport  Port=2
  Demux1 : Demux  Outputs=3
  Demux2 : Demux  Outputs=3
  Mux : Mux  Inputs=3
  Product{,1..5} (6 alike) : Product  SaturateOnIntegerOverflow=on  RndMeth=Zero  InputSameDT=on  OutDataTypeStr=Inherit: Same as first input
  Sum : Sum  Inputs=+-  SaturateOnIntegerOverflow=on  InputSameDT=on  OutDataTypeStr=Inherit: Same as first input
  Sum1 : Sum  Inputs=+-  SaturateOnIntegerOverflow=on  InputSameDT=on  OutDataTypeStr=Inherit: Same as first input
  Sum2 : Sum  Inputs=+-  SaturateOnIntegerOverflow=on  InputSameDT=on  OutDataTypeStr=Inherit: Same as first input
  u1xu2 : Outport  InitialOutput=0
  wires:
  u2/1 -> Demux1/1
  u1/1 -> Demux2/1
  Mux/1 -> u1xu2/1
  Product/1 -> Sum/1
  Product1/1 -> Sum/2
  Product2/1 -> Sum1/1
  Product3/1 -> Sum1/2
  Product4/1 -> Sum2/1
  Product5/1 -> Sum2/2
  Demux2/3 -> Product1/1, Product2/1
  Demux1/3 -> Product/2, Product3/2
  Demux2/1 -> Product3/1, Product4/1
  Demux1/2 -> Product1/2, Product4/2
  Demux2/2 -> Product/1, Product5/1
  Demux1/1 -> Product2/2, Product5/2
  Sum/1 -> Mux/1
  Sum1/1 -> Mux/2
  Sum2/1 -> Mux/3

== system newQuatLib/quat2W/quat product ==
  q1 : Inport
  q2 : Inport  Port=2
  Cross Product : Subsystem  Tag=68  mask(CrossProduct){}
      mask help: Compute the cross product of two 3-vectors : y = u1 x u2
      mask Display:
      | plot([.4 .6],[.4 .6]);
      | plot([.6 .4],[.4 .6]);
  Demux : Demux  Outputs=[1 3]
  Demux1 : Demux  Outputs=[1 3]
  Dot Product : DotProduct  InputSameDT=on  OutDataTypeStr=Inherit: Inherit via internal rule
  Mux : Mux  Inputs=2
  Product : Product  SaturateOnIntegerOverflow=on  OutDataTypeStr=Inherit: Same as first input
  Product1 : Product  SaturateOnIntegerOverflow=on  OutDataTypeStr=Inherit: Same as first input
  Product2 : Product  SaturateOnIntegerOverflow=on  OutDataTypeStr=Inherit: Same as first input
  Sum : Sum  Inputs=+++  SaturateOnIntegerOverflow=on
  Sum1 : Sum  Inputs=|+-  SaturateOnIntegerOverflow=on
  q1*q2 : Outport
  wires:
  Demux/2 -> Product1/2, Cross Product/1(u1), Dot Product/2
  Demux/1 -> Product/1, Product2/1
  Demux1/1 -> Product1/1, Product2/2
  Demux1/2 -> Cross Product/2(u2), Product/2, Dot Product/1
  Cross Product/1(u1xu2) -> Sum/2
  Product/1 -> Sum/1
  Product1/1 -> Sum/3
  Sum/1 -> Mux/2  "vector"
  Product2/1 -> Sum1/1
  Dot Product/1 -> Sum1/2
  Sum1/1 -> Mux/1  "scalar"
  q1/1 -> Demux/1
  Mux/1 -> q1*q2/1
  q2/1 -> Demux1/1

== system newQuatLib/quat2W/transposeQuaternion ==
  q : Inport
  Gain1 : Gain  Gain=[1 -1 -1 -1]  SaturateOnIntegerOverflow=on  OutDataTypeStr=Inherit: Same as input  ParamDataTypeStr=Inherit: Same as input
  q' : Outport
  wires:
  q/1 -> Gain1/1
  Gain1/1 -> q'/1

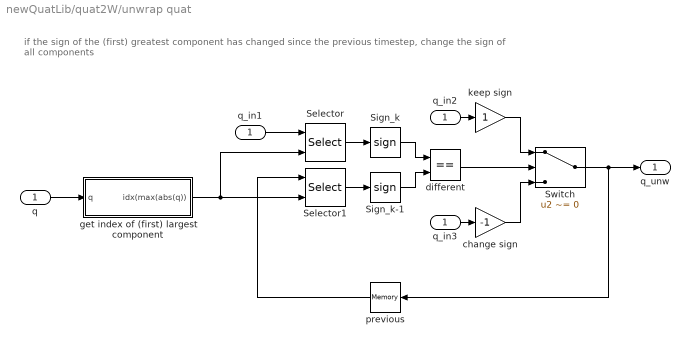
== system newQuatLib/quat2W/unwrap quat ==
  note: if the sign of the (first) greatest component has changed since the previous timestep, change the sign of all components
  q : Inport
  Selector : Selector  InputPortWidth=4  IndexOptions=Index vector (port)  Indices=[1 3]
  Selector1 : Selector  InputPortWidth=4  IndexOptions=Index vector (port)  Indices=[1 3]
  Sign_k : Signum
  Sign_k-1 : Signum
  Switch : Switch  Criteria=u2 ~= 0
  change sign : Gain  Gain=-1
  different : RelationalOperator  Operator===  OutDataTypeStr=boolean
  get index of (first) largest component : Subsystem
  keep sign : Gain
  previous : Memory  X0=[1 1 1 1]  InheritSampleTime=on
  q_in1 : InportShadow
  q_in2 : InportShadow
  q_in3 : InportShadow
  q_unw : Outport
  wires:
  q_in3/1 -> change sign/1
  change sign/1 -> Switch/3
  keep sign/1 -> Switch/1
  q_in2/1 -> keep sign/1
  different/1 -> Switch/2
  Sign_k/1 -> different/1
  Sign_k-1/1 -> different/2
  Selector/1 -> Sign_k/1
  q_in1/1 -> Selector/1
  Switch/1 -> q_unw/1, previous/1
  previous/1 -> Selector1/1
  Selector1/1 -> Sign_k-1/1
  get index of (first) largest component/1(idx(max(abs(q))) -> Selector/2, Selector1/2
  q/1 -> get index of (first) largest component/1(q)

== system newQuatLib/quat2rot/Norm ==
  X : Inport
  Dot Product1 : DotProduct  InputSameDT=on  OutDataTypeStr=Inherit: Inherit via internal rule
  Math Function : Math  Operator=sqrt  SaturateOnIntegerOverflow=on
  ||X|| : Outport  InitialOutput=0
  wires:
  Math Function/1 -> ||X||/1
  Dot Product1/1 -> Math Function/1
  X/1 -> Dot Product1/2, Dot Product1/1

== system newQuatLib/random isotropic quaternion/Normalization ==
  X : Inport
      settings: AttributesFormatString=(#%<Tag>)
      mask Help: eval('AstrolibHelp');
  Constant : Constant
  Norm : Subsystem  mask(Norm){}
      mask help: Computes the norm of a vector : y = ||u||.
      settings: AttributesFormatString=(#%<Tag>)
      mask Help: eval('AstrolibHelp');
      mask Display: disp('||X||');
  Product : Product  Inputs=*/  RndMeth=Zero
  avoid div by zero : Switch  Criteria=u2 ~= 0
  x(1) = 1 : Assignment  DiagnosticForDimensions=Warning
  X/||X|| : Outport  InitialOutput=0
      settings: AttributesFormatString=(#%<Tag>)
      mask Help: eval('AstrolibHelp');
  wires:
  Norm/1(||X||) -> Product/2, avoid div by zero/2
  X/1 -> Product/1, x(1) = 1/1, Norm/1(X)
  Product/1 -> avoid div by zero/1
  avoid div by zero/1 -> X/||X||/1
  x(1) = 1/1 -> avoid div by zero/3
  Constant/1 -> x(1) = 1/2

== system newQuatLib/unwrap quat/get index of (first) largest component ==
  q : Inport
  Abs : Abs
  Relational Operator : RelationalOperator  Operator===
  discriminate : Gain  Gain=[1 2 3 4]
  double : DataTypeConversion  OutDataTypeStr=double
  find : MinMax  Function=max
  max : MinMax  Function=max
  idx(max(abs(q)) : Outport
  wires:
  double/1 -> discriminate/1
  discriminate/1 -> find/1
  q/1 -> Abs/1
  Abs/1 -> max/1, Relational Operator/1
  max/1 -> Relational Operator/2
  Relational Operator/1 -> double/1  "1 for the greatest component(s)"
  find/1 -> idx(max(abs(q))/1  "index of first greatest component"

== system newQuatLib/vects2frame/Normalization ==
  X : Inport
      settings: AttributesFormatString=(#%<Tag>)
      mask Help: eval('AstrolibHelp');
  Constant : Constant
  Norm : Subsystem  mask(Norm){}
      mask help: Computes the norm of a vector : y = ||u||.
      settings: AttributesFormatString=(#%<Tag>)
      mask Help: eval('AstrolibHelp');
      mask Display: disp('||X||');
  Product : Product  Inputs=*/  RndMeth=Zero
  avoid div by zero : Switch  Criteria=u2 ~= 0
  x(1) = 1 : Assignment  DiagnosticForDimensions=Warning
  X/||X|| : Outport  InitialOutput=0
      settings: AttributesFormatString=(#%<Tag>)
      mask Help: eval('AstrolibHelp');
  wires:
  Constant/1 -> x(1) = 1/2
  x(1) = 1/1 -> avoid div by zero/3
  avoid div by zero/1 -> X/||X||/1
  Product/1 -> avoid div by zero/1
  X/1 -> Norm/1(X), x(1) = 1/1, Product/1
  Norm/1(||X||) -> avoid div by zero/2, Product/2

== system newQuatLib/vects2frame/Normalization1 ==
  X : Inport
      settings: AttributesFormatString=(#%<Tag>)
      mask Help: eval('AstrolibHelp');
  Constant : Constant
  Norm : Subsystem  mask(Norm){}
      mask help: Computes the norm of a vector : y = ||u||.
      settings: AttributesFormatString=(#%<Tag>)
      mask Help: eval('AstrolibHelp');
      mask Display: disp('||X||');
  Product : Product  Inputs=*/  RndMeth=Zero
  avoid div by zero : Switch  Criteria=u2 ~= 0
  x(1) = 1 : Assignment  DiagnosticForDimensions=Warning
  X/||X|| : Outport  InitialOutput=0
      settings: AttributesFormatString=(#%<Tag>)
      mask Help: eval('AstrolibHelp');
  wires:
  Norm/1(||X||) -> Product/2, avoid div by zero/2
  X/1 -> Product/1, x(1) = 1/1, Norm/1(X)
  Product/1 -> avoid div by zero/1
  avoid div by zero/1 -> X/||X||/1
  x(1) = 1/1 -> avoid div by zero/3
  Constant/1 -> x(1) = 1/2

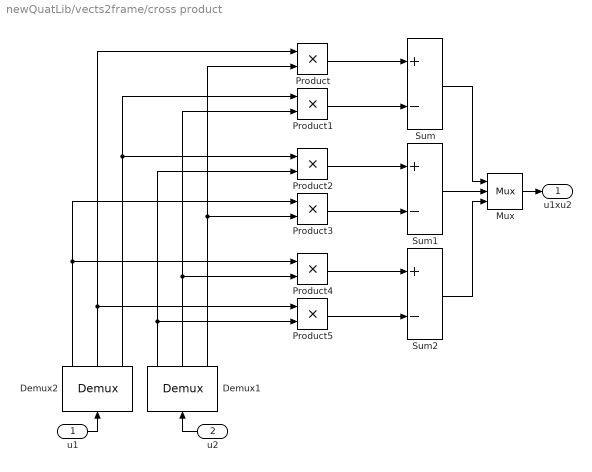
== system newQuatLib/vects2frame/cross product ==
  u1 : Inport  PortDimensions=3
  u2 : Inport  Port=2  PortDimensions=3
  Demux1 : Demux  Outputs=3
  Demux2 : Demux  Outputs=3
  Mux : Mux  Inputs=3
  Product{,1..5} (6 alike) : Product  SaturateOnIntegerOverflow=on  RndMeth=Zero  InputSameDT=on  OutDataTypeStr=Inherit: Same as first input
  Sum : Sum  Inputs=+-  SaturateOnIntegerOverflow=on  InputSameDT=on  OutDataTypeStr=Inherit: Same as first input
  Sum1 : Sum  Inputs=+-  SaturateOnIntegerOverflow=on  InputSameDT=on  OutDataTypeStr=Inherit: Same as first input
  Sum2 : Sum  Inputs=+-  SaturateOnIntegerOverflow=on  InputSameDT=on  OutDataTypeStr=Inherit: Same as first input
  u1xu2 : Outport  PortDimensions=3  InitialOutput=0
  wires:
  u2/1 -> Demux1/1
  u1/1 -> Demux2/1
  Mux/1 -> u1xu2/1
  Product/1 -> Sum/1
  Product1/1 -> Sum/2
  Product2/1 -> Sum1/1
  Product3/1 -> Sum1/2
  Product4/1 -> Sum2/1
  Product5/1 -> Sum2/2
  Demux2/3 -> Product1/1, Product2/1
  Demux1/3 -> Product/2, Product3/2
  Demux2/1 -> Product3/1, Product4/1
  Demux1/2 -> Product1/2, Product4/2
  Demux2/2 -> Product/1, Product5/1
  Demux1/1 -> Product2/2, Product5/2
  Sum/1 -> Mux/1
  Sum1/1 -> Mux/2
  Sum2/1 -> Mux/3

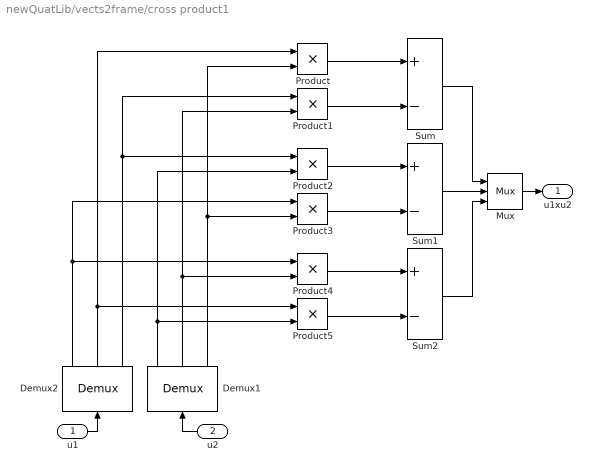
== system newQuatLib/vects2frame/cross product1 ==
  u1 : Inport  PortDimensions=3
  u2 : Inport  Port=2  PortDimensions=3
  Demux1 : Demux  Outputs=3
  Demux2 : Demux  Outputs=3
  Mux : Mux  Inputs=3
  Product{,1..5} (6 alike) : Product  SaturateOnIntegerOverflow=on  RndMeth=Zero  InputSameDT=on  OutDataTypeStr=Inherit: Same as first input
  Sum : Sum  Inputs=+-  SaturateOnIntegerOverflow=on  InputSameDT=on  OutDataTypeStr=Inherit: Same as first input
  Sum1 : Sum  Inputs=+-  SaturateOnIntegerOverflow=on  InputSameDT=on  OutDataTypeStr=Inherit: Same as first input
  Sum2 : Sum  Inputs=+-  SaturateOnIntegerOverflow=on  InputSameDT=on  OutDataTypeStr=Inherit: Same as first input
  u1xu2 : Outport  PortDimensions=3  InitialOutput=0
  wires:
  Sum2/1 -> Mux/3
  Sum1/1 -> Mux/2
  Sum/1 -> Mux/1
  Demux1/1 -> Product5/2, Product2/2
  Demux2/2 -> Product5/1, Product/1
  Demux1/2 -> Product4/2, Product1/2
  Demux2/1 -> Product4/1, Product3/1
  Demux1/3 -> Product3/2, Product/2
  Demux2/3 -> Product2/1, Product1/1
  Product5/1 -> Sum2/2
  Product4/1 -> Sum2/1
  Product3/1 -> Sum1/2
  Product2/1 -> Sum1/1
  Product1/1 -> Sum/2
  Product/1 -> Sum/1
  Mux/1 -> u1xu2/1
  u1/1 -> Demux2/1
  u2/1 -> Demux1/1

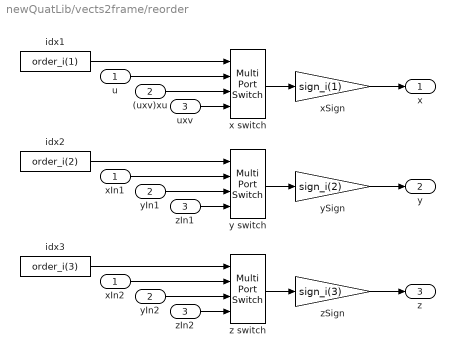
== system newQuatLib/vects2frame/reorder ==
  u : Inport
  (uxv)xu : Inport  Port=2
  uxv : Inport  Port=3
  idx1 : Constant  Value=order_i(1)
  idx2 : Constant  Value=order_i(2)
  idx3 : Constant  Value=order_i(3)
  x switch : MultiPortSwitch
  xIn1 : InportShadow
  xIn2 : InportShadow
  xSign : Gain  Gain=sign_i(1)
  y switch : MultiPortSwitch
  yIn1 : InportShadow  Port=2
  yIn2 : InportShadow  Port=2
  ySign : Gain  Gain=sign_i(2)
  z switch : MultiPortSwitch
  zIn1 : InportShadow  Port=3
  zIn2 : InportShadow  Port=3
  zSign : Gain  Gain=sign_i(3)
  x : Outport
  y : Outport  Port=2
  z : Outport  Port=3
  wires:
  xIn1/1 -> y switch/2
  yIn1/1 -> y switch/3
  zIn1/1 -> y switch/4
  xIn2/1 -> z switch/2
  yIn2/1 -> z switch/3
  zIn2/1 -> z switch/4
  uxv/1 -> x switch/4
  (uxv)xu/1 -> x switch/3
  u/1 -> x switch/2
  xSign/1 -> x/1
  z switch/1 -> zSign/1
  idx1/1 -> x switch/1
  x switch/1 -> xSign/1
  y switch/1 -> ySign/1
  idx2/1 -> y switch/1
  idx3/1 -> z switch/1
  ySign/1 -> y/1
  zSign/1 -> z/1

== system newQuatLib/W2Quat/Normalization/Norm ==
  X : Inport
  Dot Product1 : DotProduct  InputSameDT=on  OutDataTypeStr=Inherit: Inherit via internal rule
  Math Function : Math  Operator=sqrt  SaturateOnIntegerOverflow=on
  ||X|| : Outport  InitialOutput=0
  wires:
  Math Function/1 -> ||X||/1
  Dot Product1/1 -> Math Function/1
  X/1 -> Dot Product1/2, Dot Product1/1

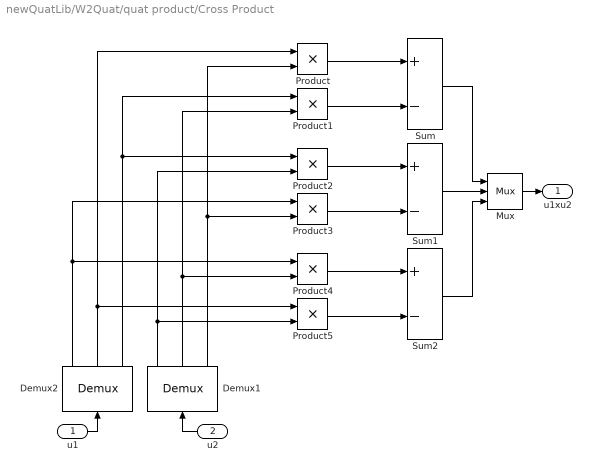
== system newQuatLib/W2Quat/quat product/Cross Product ==
  u1 : Inport
  u2 : Inport  Port=2
  Demux1 : Demux  Outputs=3
  Demux2 : Demux  Outputs=3
  Mux : Mux  Inputs=3
  Product{,1..5} (6 alike) : Product  SaturateOnIntegerOverflow=on  RndMeth=Zero  InputSameDT=on  OutDataTypeStr=Inherit: Same as first input
  Sum : Sum  Inputs=+-  SaturateOnIntegerOverflow=on  InputSameDT=on  OutDataTypeStr=Inherit: Same as first input
  Sum1 : Sum  Inputs=+-  SaturateOnIntegerOverflow=on  InputSameDT=on  OutDataTypeStr=Inherit: Same as first input
  Sum2 : Sum  Inputs=+-  SaturateOnIntegerOverflow=on  InputSameDT=on  OutDataTypeStr=Inherit: Same as first input
  u1xu2 : Outport  InitialOutput=0
  wires:
  u2/1 -> Demux1/1
  u1/1 -> Demux2/1
  Mux/1 -> u1xu2/1
  Product/1 -> Sum/1
  Product1/1 -> Sum/2
  Product2/1 -> Sum1/1
  Product3/1 -> Sum1/2
  Product4/1 -> Sum2/1
  Product5/1 -> Sum2/2
  Demux2/3 -> Product1/1, Product2/1
  Demux1/3 -> Product/2, Product3/2
  Demux2/1 -> Product3/1, Product4/1
  Demux1/2 -> Product1/2, Product4/2
  Demux2/2 -> Product/1, Product5/1
  Demux1/1 -> Product2/2, Product5/2
  Sum/1 -> Mux/1
  Sum1/1 -> Mux/2
  Sum2/1 -> Mux/3

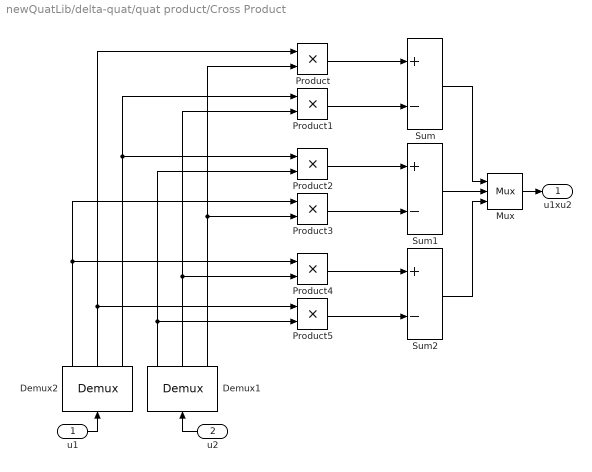
== system newQuatLib/delta-quat/quat product/Cross Product ==
  u1 : Inport
  u2 : Inport  Port=2
  Demux1 : Demux  Outputs=3
  Demux2 : Demux  Outputs=3
  Mux : Mux  Inputs=3
  Product{,1..5} (6 alike) : Product  SaturateOnIntegerOverflow=on  RndMeth=Zero  InputSameDT=on  OutDataTypeStr=Inherit: Same as first input
  Sum : Sum  Inputs=+-  SaturateOnIntegerOverflow=on  InputSameDT=on  OutDataTypeStr=Inherit: Same as first input
  Sum1 : Sum  Inputs=+-  SaturateOnIntegerOverflow=on  InputSameDT=on  OutDataTypeStr=Inherit: Same as first input
  Sum2 : Sum  Inputs=+-  SaturateOnIntegerOverflow=on  InputSameDT=on  OutDataTypeStr=Inherit: Same as first input
  u1xu2 : Outport  InitialOutput=0
  wires:
  u2/1 -> Demux1/1
  u1/1 -> Demux2/1
  Mux/1 -> u1xu2/1
  Product/1 -> Sum/1
  Product1/1 -> Sum/2
  Product2/1 -> Sum1/1
  Product3/1 -> Sum1/2
  Product4/1 -> Sum2/1
  Product5/1 -> Sum2/2
  Demux2/3 -> Product1/1, Product2/1
  Demux1/3 -> Product/2, Product3/2
  Demux2/1 -> Product3/1, Product4/1
  Demux1/2 -> Product1/2, Product4/2
  Demux2/2 -> Product/1, Product5/1
  Demux1/1 -> Product2/2, Product5/2
  Sum/1 -> Mux/1
  Sum1/1 -> Mux/2
  Sum2/1 -> Mux/3

== system newQuatLib/eurl2quat (small angles)/Normalization/Norm ==
  X : Inport
  Dot Product1 : DotProduct  InputSameDT=on  OutDataTypeStr=Inherit: Inherit via internal rule
  Math Function : Math  Operator=sqrt  SaturateOnIntegerOverflow=on
  ||X|| : Outport  InitialOutput=0
  wires:
  Math Function/1 -> ||X||/1
  Dot Product1/1 -> Math Function/1
  X/1 -> Dot Product1/2, Dot Product1/1

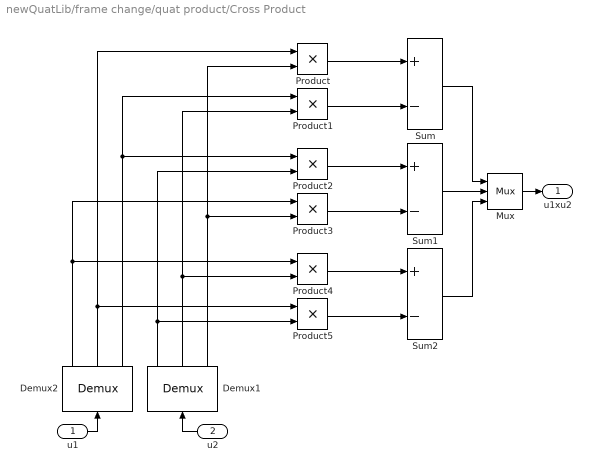
== system newQuatLib/frame change/quat product/Cross Product ==
  u1 : Inport
  u2 : Inport  Port=2
  Demux1 : Demux  Outputs=3
  Demux2 : Demux  Outputs=3
  Mux : Mux  Inputs=3
  Product{,1..5} (6 alike) : Product  SaturateOnIntegerOverflow=on  RndMeth=Zero  InputSameDT=on  OutDataTypeStr=Inherit: Same as first input
  Sum : Sum  Inputs=+-  SaturateOnIntegerOverflow=on  InputSameDT=on  OutDataTypeStr=Inherit: Same as first input
  Sum1 : Sum  Inputs=+-  SaturateOnIntegerOverflow=on  InputSameDT=on  OutDataTypeStr=Inherit: Same as first input
  Sum2 : Sum  Inputs=+-  SaturateOnIntegerOverflow=on  InputSameDT=on  OutDataTypeStr=Inherit: Same as first input
  u1xu2 : Outport  InitialOutput=0
  wires:
  u2/1 -> Demux1/1
  u1/1 -> Demux2/1
  Mux/1 -> u1xu2/1
  Product/1 -> Sum/1
  Product1/1 -> Sum/2
  Product2/1 -> Sum1/1
  Product3/1 -> Sum1/2
  Product4/1 -> Sum2/1
  Product5/1 -> Sum2/2
  Demux2/3 -> Product1/1, Product2/1
  Demux1/3 -> Product/2, Product3/2
  Demux2/1 -> Product3/1, Product4/1
  Demux1/2 -> Product1/2, Product4/2
  Demux2/2 -> Product/1, Product5/1
  Demux1/1 -> Product2/2, Product5/2
  Sum/1 -> Mux/1
  Sum1/1 -> Mux/2
  Sum2/1 -> Mux/3
